simulink model "torquelimiter"  (R2024b)
settings: Solver=FixedStepAuto  StartTime=0.0  StopTime=inf  FixedStep=0.001  RelTol=1e-3
settings Model: Creator=kara.28  LastModifiedBy=kara.28

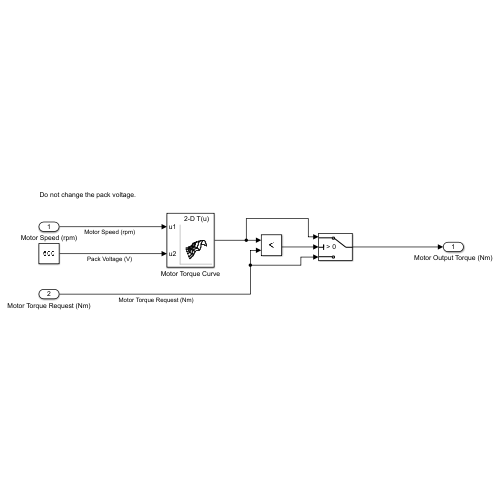
[thumbnail: Simulink's stored preview of the top-level diagram]
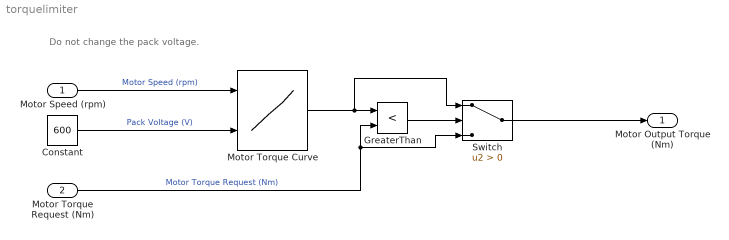
== system torquelimiter ==
  note: Do not change the pack voltage.
  Motor Speed (rpm) : Inport
  Motor Torque Request (Nm) : Inport  Port=2
  Constant : Constant  Value=600
  GreaterThan : RelationalOperator  Operator=<  OutDataTypeStr=boolean  RndMeth=Simplest  InputSameDT=off
  Motor Torque Curve : Lookup_n-D  BreakpointsForDimension1=[0;2000;4000;6000;8000;10000;12000;13000;14000;16000;18000;19000]  BreakpointsForDimension2=[500;600]  BreakpointsForDimension3=[500, 600]  Table=[13.93365 21.184926180000001;12.71866 21.107310760000001;11.85909 21.171799480000001;11.354939999999999 21.165465080000001;10.70875 21.23010644;10.204750000000001 21.152643659999999;9.5584880000000005 21.217132379999999;9.4130249999999993 21.214003340000001;9.1965109999999992 19.93109755;8.6212260000000001 15.51709269;8.04617 8.0461698530000003;0 0]  InterpMethod=Cubic spline  ExtrapMethod=Clip  InternalRulePriority=Speed  RndMeth=Simplest
      settings: InputPortMap=u0,u1
  Switch : Switch  Criteria=u2 > Threshold  SaturateOnIntegerOverflow=off  InputSameDT=off
  Motor Output Torque (Nm) : Outport
  wires:
  Motor Torque Curve/1 -> Switch/1, GreaterThan/1
  GreaterThan/1 -> Switch/2
  Motor Torque Request (Nm)/1 -> Switch/3, GreaterThan/2  "Motor Torque Request (Nm)"
  Constant/1 -> Motor Torque Curve/2  "Pack Voltage (V)"
  Switch/1 -> Motor Output Torque (Nm)/1
  Motor Speed (rpm)/1 -> Motor Torque Curve/1  "Motor Speed (rpm)"
